simulink model "sen"  (R2017b)
settings: Solver=VariableStepAuto  StartTime=0.0  StopTime=10.0  RelTol=1e-3
libraries: fuzblock x1, simulink x1
settings Model: Creator=Estudiantes  LastModifiedBy=Estudiantes

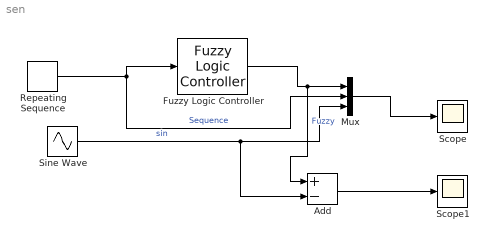
== system sen ==
  Add : Sum  Inputs=+-
  Fuzzy Logic Controller : fuzblock/Fuzzy Logic  Controller  FIS=sistemats  OutputSampleNumber=101  DataType=double  FuzzifiedInputs=off  RuleFiringStrengths=off  RuleOutputs=off  AggregatedOutputs=off  SimulateUsing=Interpreted execution
  Mux : Mux  Inputs=3
  Repeating Sequence : simulink/Sources/Repeating Sequence  rep_seq_t=[0 1 2 3 4]  rep_seq_y="[0  1 0 -1 0]"
  Scope : Scope
  Scope1 : Scope
  Sine Wave : Sin  Phase=2*pi/4  SampleTime=0
  wires:
  Mux/1 -> Scope/1
  Fuzzy Logic Controller/1 -> Add/1, Mux/1  "Fuzzy"
  Repeating Sequence/1 -> Mux/2, Fuzzy Logic Controller/1  "Sequence"
  Sine Wave/1 -> Add/2, Mux/3  "sin"
  Add/1 -> Scope1/1
